simulink model "Quad_Nonlinear_Roll_PS"  (R2023a)
settings: Solver=ode4  StartTime=0.0  StopTime=0.5  FixedStep=0.02  RelTol=1e-3
values from neighbouring files (symbols this model uses):
  b = 1.10794e-5    (= 1.10794e-05)    [QuadParameter.m]    (also in Scenario_I.mat = 3.13e-05; Scenario_II.mat = 3.13e-05; final_PS.m = 3.6602e-06)
  d = 3.2e-6    (= 3.2e-06)    [QuadParameter.m]    (also in Scenario_I.mat; Scenario_II.mat)
  d_cg = 0.295    [QuadParameter.m]
  Gamma1 = Ixz*(Ixx - Iyy + Izz)/Gamma    [QuadConstants_v1.m]    (also in final_PS.m = 4.98954110218e-06)
  Gamma10 = (Ixx - Iyy)*Ixx + Ixz^2/Gamma    [QuadConstants_v1.m]    (also in final_PS.m = -1.44562619786e-05)
  Gamma11 = Ixx/Gamma    [QuadConstants_v1.m]    (also in final_PS.m = 24.4566929368)
  Gamma2 = Izz*(Izz - Iyy) + Ixz^2    [QuadConstants_v1.m]    (also in final_PS.m = 0.00290613207976)
  Gamma3 = Izz/Gamma    [QuadConstants_v1.m]    (also in final_PS.m = 42.1805100768)
  Gamma4 = Ixz/Gamma    [QuadConstants_v1.m]    (also in final_PS.m = 0.000237183411278)
  Gamma5 = I_rotor/Ixx    [QuadConstants_v1.m]    (also in final_PS.m = -0.0023457751623)
  Gamma6 = (Izz - Ixx)/Iyy    [QuadConstants_v1.m]    (also in final_PS.m = 2.52935414321)
  Gamma8 = 1/Iyy    [QuadConstants_v1.m]    (also in final_PS.m = 18.4688604257)
  Gamma9 = I_rotor/Iyy    [QuadConstants_v1.m]    (also in final_PS.m = 0.00216966508126)
  init_I = data(1, :)    [load_data.m]
  init_II = data(1, :)    [load_data.m]
  init_III = data(1, :)    [load_data.m]
  init_IV = data(1, :)    [load_data.m]
  init_V = data(1, :)    [load_data.m]
  Omega_I = Omega    [load_data.m]
  Omega_II = Omega    [load_data.m]
  Omega_III = Omega    [load_data.m]
  Omega_IV = Omega    [load_data.m]
  Omega_V = Omega    [load_data.m]
(part 1 of 2)
settings Model: Creator=Ali  LastModifiedBy=Ali
settings SolverCC: AlgebraicLoopSolver=TrustRegion
settings DebuggingCC: UnconnectedInputMsg=warning  UnconnectedOutputMsg=warning  UnconnectedLineMsg=warning
settings ModelReferenceCC: EnableRefExpFcnMdlSchedulingChecks=on

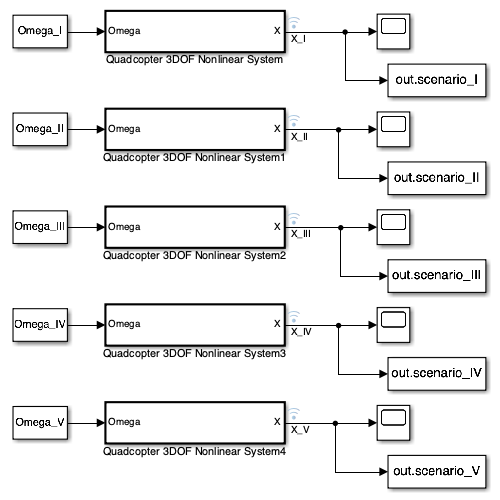
[thumbnail: Simulink's stored preview of the top-level diagram]
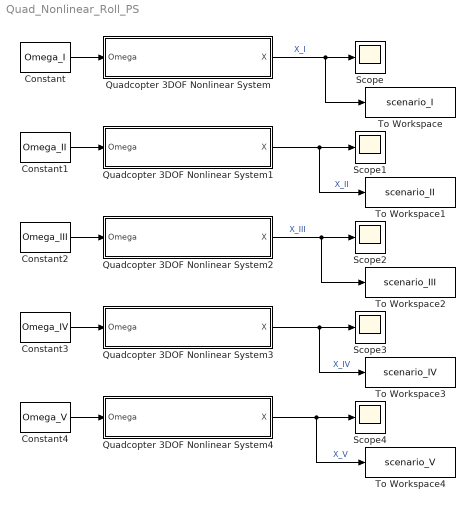
== system Quad_Nonlinear_Roll_PS ==
  Constant : Constant  Value=Omega_I
  Constant1 : Constant  Value=Omega_II
  Constant2 : Constant  Value=Omega_III
  Constant3 : Constant  Value=Omega_IV
  Constant4 : Constant  Value=Omega_V
  Quadcopter 3DOF Nonlinear System : Subsystem  TreatAsAtomicUnit=on
  Quadcopter 3DOF Nonlinear System1 : Subsystem  TreatAsAtomicUnit=on
  Quadcopter 3DOF Nonlinear System2 : Subsystem  TreatAsAtomicUnit=on
  Quadcopter 3DOF Nonlinear System3 : Subsystem  TreatAsAtomicUnit=on
  Quadcopter 3DOF Nonlinear System4 : Subsystem  TreatAsAtomicUnit=on
  Scope{,1..4} (5 alike) : Scope
  To Workspace : ToWorkspace  VariableName=scenario_I  SampleTime=-1
  To Workspace1 : ToWorkspace  VariableName=scenario_II  SampleTime=-1
  To Workspace2 : ToWorkspace  VariableName=scenario_III  SampleTime=-1
  To Workspace3 : ToWorkspace  VariableName=scenario_IV  SampleTime=-1
  To Workspace4 : ToWorkspace  VariableName=scenario_V  SampleTime=-1
  wires:
  Constant/1 -> Quadcopter 3DOF Nonlinear System/1(Omega)
  Quadcopter 3DOF Nonlinear System/1(X) -> To Workspace/1, Scope/1  "X_I"
  Quadcopter 3DOF Nonlinear System1/1(X) -> To Workspace1/1, Scope1/1  "X_II"
  Constant1/1 -> Quadcopter 3DOF Nonlinear System1/1(Omega)
  Quadcopter 3DOF Nonlinear System2/1(X) -> To Workspace2/1, Scope2/1  "X_III"
  Constant2/1 -> Quadcopter 3DOF Nonlinear System2/1(Omega)
  Quadcopter 3DOF Nonlinear System3/1(X) -> To Workspace3/1, Scope3/1  "X_IV"
  Constant3/1 -> Quadcopter 3DOF Nonlinear System3/1(Omega)
  Quadcopter 3DOF Nonlinear System4/1(X) -> To Workspace4/1, Scope4/1  "X_V"
  Constant4/1 -> Quadcopter 3DOF Nonlinear System4/1(Omega)

== system Quad_Nonlinear_Roll_PS/Quadcopter 3DOF Nonlinear System ==
  Omega : Inport
  Integrator : Integrator  InitialCondition=init_I
  Quad System : Subsystem
  X : Outport
  wires:
  Integrator/1 -> Quad System/1(X), X/1  "X"
  Quad System/1(dot(X)) -> Integrator/1  "dot(X)"
  Omega/1 -> Quad System/2(Omega)

== system Quad_Nonlinear_Roll_PS/Quadcopter 3DOF Nonlinear System1 ==
  Omega : Inport
  Integrator : Integrator  InitialCondition=init_II
  Quad System : Subsystem
  X : Outport
  wires:
  Integrator/1 -> Quad System/1(X), X/1  "X"
  Quad System/1(dot(X)) -> Integrator/1  "dot(X)"
  Omega/1 -> Quad System/2(Omega)

== system Quad_Nonlinear_Roll_PS/Quadcopter 3DOF Nonlinear System2 ==
  Omega : Inport
  Integrator : Integrator  InitialCondition=init_III
  Quad System : Subsystem
  X : Outport
  wires:
  Integrator/1 -> Quad System/1(X), X/1  "X"
  Quad System/1(dot(X)) -> Integrator/1  "dot(X)"
  Omega/1 -> Quad System/2(Omega)

== system Quad_Nonlinear_Roll_PS/Quadcopter 3DOF Nonlinear System3 ==
  Omega : Inport
  Integrator : Integrator  InitialCondition=init_IV
  Quad System : Subsystem
  X : Outport
  wires:
  Integrator/1 -> Quad System/1(X), X/1  "X"
  Quad System/1(dot(X)) -> Integrator/1  "dot(X)"
  Omega/1 -> Quad System/2(Omega)

== system Quad_Nonlinear_Roll_PS/Quadcopter 3DOF Nonlinear System4 ==
  Omega : Inport
  Integrator : Integrator  InitialCondition=init_V
  Quad System : Subsystem
  X : Outport
  wires:
  Integrator/1 -> Quad System/1(X), X/1  "X"
  Quad System/1(dot(X)) -> Integrator/1  "dot(X)"
  Omega/1 -> Quad System/2(Omega)

== system Quad_Nonlinear_Roll_PS/Quadcopter 3DOF Nonlinear System/Quad System ==
  X : Inport
  Omega : Inport  Port=2
  Quad System : Subsystem
  Selector : Selector  InputPortWidth=6  IndexOptions=Index vector (dialog)  Indices=[1 4]  OutputSizes=1
  Subsystem : Subsystem
  dot(X) : Outport
  wires:
  Selector/1 -> dot(X)/1  "dot(X)"
  X/1 -> Subsystem/1(X)
  Omega/1 -> Quad System/2(Omega)
  Quad System/1(dot(X)) -> Selector/1  "dot(X)"
  Subsystem/1(X_6) -> Quad System/1(X)

== system Quad_Nonlinear_Roll_PS/Quadcopter 3DOF Nonlinear System1/Quad System ==
  X : Inport
  Omega : Inport  Port=2
  Quad System : Subsystem
  Selector : Selector  InputPortWidth=6  IndexOptions=Index vector (dialog)  Indices=[1 4]  OutputSizes=1
  Subsystem : Subsystem
  dot(X) : Outport
  wires:
  Selector/1 -> dot(X)/1  "dot(X)"
  X/1 -> Subsystem/1(X)
  Omega/1 -> Quad System/2(Omega)
  Quad System/1(dot(X)) -> Selector/1  "dot(X)"
  Subsystem/1(X_6) -> Quad System/1(X)

== system Quad_Nonlinear_Roll_PS/Quadcopter 3DOF Nonlinear System2/Quad System ==
  X : Inport
  Omega : Inport  Port=2
  Quad System : Subsystem
  Selector : Selector  InputPortWidth=6  IndexOptions=Index vector (dialog)  Indices=[1 4]  OutputSizes=1
  Subsystem : Subsystem
  dot(X) : Outport
  wires:
  Selector/1 -> dot(X)/1  "dot(X)"
  X/1 -> Subsystem/1(X)
  Omega/1 -> Quad System/2(Omega)
  Quad System/1(dot(X)) -> Selector/1  "dot(X)"
  Subsystem/1(X_6) -> Quad System/1(X)

== system Quad_Nonlinear_Roll_PS/Quadcopter 3DOF Nonlinear System3/Quad System ==
  X : Inport
  Omega : Inport  Port=2
  Quad System : Subsystem
  Selector : Selector  InputPortWidth=6  IndexOptions=Index vector (dialog)  Indices=[1 4]  OutputSizes=1
  Subsystem : Subsystem
  dot(X) : Outport
  wires:
  Selector/1 -> dot(X)/1  "dot(X)"
  X/1 -> Subsystem/1(X)
  Omega/1 -> Quad System/2(Omega)
  Quad System/1(dot(X)) -> Selector/1  "dot(X)"
  Subsystem/1(X_6) -> Quad System/1(X)

== system Quad_Nonlinear_Roll_PS/Quadcopter 3DOF Nonlinear System4/Quad System ==
  X : Inport
  Omega : Inport  Port=2
  Quad System : Subsystem
  Selector : Selector  InputPortWidth=6  IndexOptions=Index vector (dialog)  Indices=[1 4]  OutputSizes=1
  Subsystem : Subsystem
  dot(X) : Outport
  wires:
  Selector/1 -> dot(X)/1  "dot(X)"
  X/1 -> Subsystem/1(X)
  Omega/1 -> Quad System/2(Omega)
  Quad System/1(dot(X)) -> Selector/1  "dot(X)"
  Subsystem/1(X_6) -> Quad System/1(X)

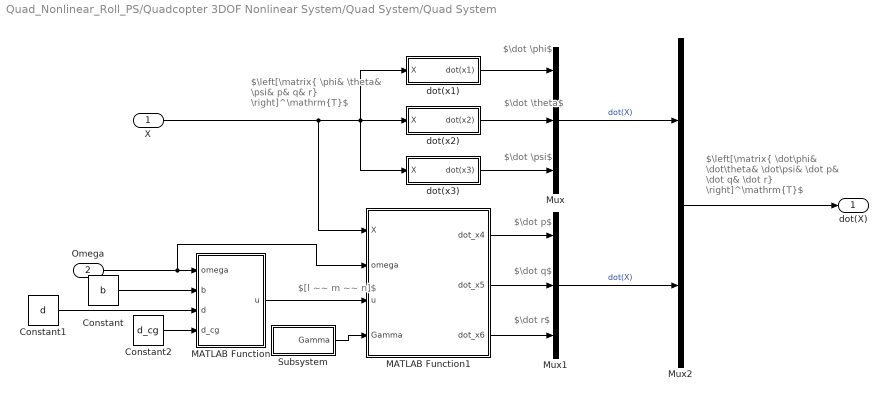
== system Quad_Nonlinear_Roll_PS/Quadcopter 3DOF Nonlinear System/Quad System/Quad System ==
  note: $\dot \phi$
  note: $\left[\matrix{ \phi& \theta& \psi& p& q& r} \right]^\mathrm{T}$
  note: $[l ~~ m ~~ n]$
  note: $\dot \theta$
  note: $\dot \psi$
  note: $\dot p$
  note: $\dot q$
  note: $\dot r$
  note: $\left[\matrix{ \dot\phi& \dot\theta& \dot\psi& \dot p& \dot q& \dot r} \right]^\mathrm{T}$
  X : Inport
  Omega : Inport  Port=2
  Constant : Constant  Value=b
  Constant1 : Constant  Value=d
  Constant2 : Constant  Value=d_cg
  MATLAB Function : MATLAB Function  TreatAsAtomicUnit=on
  MATLAB Function1 : MATLAB Function  TreatAsAtomicUnit=on
  Mux : Mux  Inputs=3
  Mux1 : Mux  Inputs=3
  Mux2 : Mux  Inputs=2
  Subsystem : Subsystem
  dot(x1) : Subsystem
  dot(x2) : Subsystem
  dot(x3) : Subsystem
  dot(X) : Outport
  wires:
  X/1 -> MATLAB Function1/1(X), dot(x3)/1(X), dot(x1)/1(X), dot(x2)/1(X)
  Omega/1 -> MATLAB Function1/2(omega), MATLAB Function/1(omega)
  MATLAB Function1/2(dot_x5) -> Mux1/2
  dot(x2)/1(dot(x2)) -> Mux/2
  MATLAB Function1/1(dot_x4) -> Mux1/1
  dot(x3)/1(dot(x3)) -> Mux/3
  dot(x1)/1(dot(x1)) -> Mux/1
  MATLAB Function1/3(dot_x6) -> Mux1/3
  Constant/1 -> MATLAB Function/2(b)
  Constant1/1 -> MATLAB Function/3(d)
  MATLAB Function/1(u) -> MATLAB Function1/3(u)
  Mux1/1 -> Mux2/2  "dot(X)"
  Mux/1 -> Mux2/1  "dot(X)"
  Mux2/1 -> dot(X)/1
  Subsystem/1(Gamma) -> MATLAB Function1/4(Gamma)
  Constant2/1 -> MATLAB Function/4(d_cg)

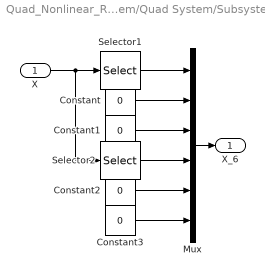
== system Quad_Nonlinear_Roll_PS/Quadcopter 3DOF Nonlinear System/Quad System/Subsystem ==
  X : Inport
  Constant{,1..3} (4 alike) : Constant  Value=0
  Mux : Mux  Inputs=6
  Selector1 : Selector  InputPortWidth=2  IndexOptions=Index vector (dialog)  Indices=[1]  OutputSizes=1
  Selector2 : Selector  InputPortWidth=2  IndexOptions=Index vector (dialog)  Indices=[2]  OutputSizes=1
  X_6 : Outport
  wires:
  Constant3/1 -> Mux/6
  Constant1/1 -> Mux/3
  Mux/1 -> X_6/1
  Constant/1 -> Mux/2
  Selector2/1 -> Mux/4
  Selector1/1 -> Mux/1
  Constant2/1 -> Mux/5
  X/1 -> Selector2/1, Selector1/1

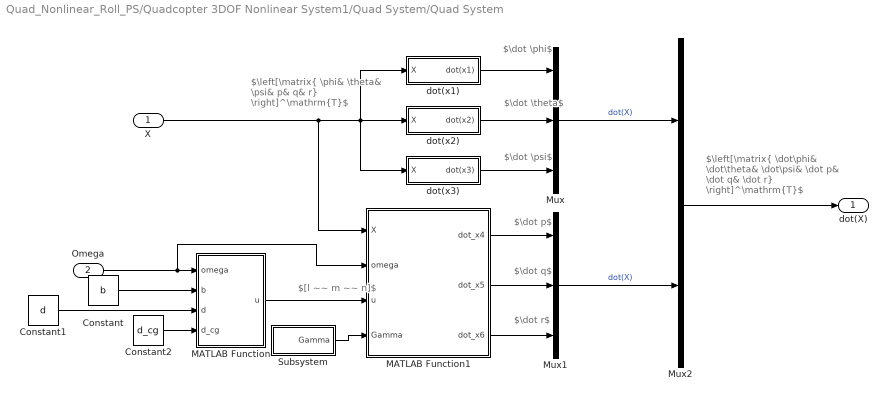
== system Quad_Nonlinear_Roll_PS/Quadcopter 3DOF Nonlinear System1/Quad System/Quad System ==
  note: $\dot \phi$
  note: $\left[\matrix{ \phi& \theta& \psi& p& q& r} \right]^\mathrm{T}$
  note: $[l ~~ m ~~ n]$
  note: $\dot \theta$
  note: $\dot \psi$
  note: $\dot p$
  note: $\dot q$
  note: $\dot r$
  note: $\left[\matrix{ \dot\phi& \dot\theta& \dot\psi& \dot p& \dot q& \dot r} \right]^\mathrm{T}$
  X : Inport
  Omega : Inport  Port=2
  Constant : Constant  Value=b
  Constant1 : Constant  Value=d
  Constant2 : Constant  Value=d_cg
  MATLAB Function : MATLAB Function  TreatAsAtomicUnit=on
  MATLAB Function1 : MATLAB Function  TreatAsAtomicUnit=on
  Mux : Mux  Inputs=3
  Mux1 : Mux  Inputs=3
  Mux2 : Mux  Inputs=2
  Subsystem : Subsystem
  dot(x1) : Subsystem
  dot(x2) : Subsystem
  dot(x3) : Subsystem
  dot(X) : Outport
  wires:
  X/1 -> MATLAB Function1/1(X), dot(x3)/1(X), dot(x1)/1(X), dot(x2)/1(X)
  Omega/1 -> MATLAB Function1/2(omega), MATLAB Function/1(omega)
  MATLAB Function1/2(dot_x5) -> Mux1/2
  dot(x2)/1(dot(x2)) -> Mux/2
  MATLAB Function1/1(dot_x4) -> Mux1/1
  dot(x3)/1(dot(x3)) -> Mux/3
  dot(x1)/1(dot(x1)) -> Mux/1
  MATLAB Function1/3(dot_x6) -> Mux1/3
  Constant/1 -> MATLAB Function/2(b)
  Constant1/1 -> MATLAB Function/3(d)
  MATLAB Function/1(u) -> MATLAB Function1/3(u)
  Mux1/1 -> Mux2/2  "dot(X)"
  Mux/1 -> Mux2/1  "dot(X)"
  Mux2/1 -> dot(X)/1
  Subsystem/1(Gamma) -> MATLAB Function1/4(Gamma)
  Constant2/1 -> MATLAB Function/4(d_cg)

== system Quad_Nonlinear_Roll_PS/Quadcopter 3DOF Nonlinear System1/Quad System/Subsystem ==
  X : Inport
  Constant{,1..3} (4 alike) : Constant  Value=0
  Mux : Mux  Inputs=6
  Selector1 : Selector  InputPortWidth=2  IndexOptions=Index vector (dialog)  Indices=[1]  OutputSizes=1
  Selector2 : Selector  InputPortWidth=2  IndexOptions=Index vector (dialog)  Indices=[2]  OutputSizes=1
  X_6 : Outport
  wires:
  Constant3/1 -> Mux/6
  Constant1/1 -> Mux/3
  Mux/1 -> X_6/1
  Constant/1 -> Mux/2
  Selector2/1 -> Mux/4
  Selector1/1 -> Mux/1
  Constant2/1 -> Mux/5
  X/1 -> Selector2/1, Selector1/1

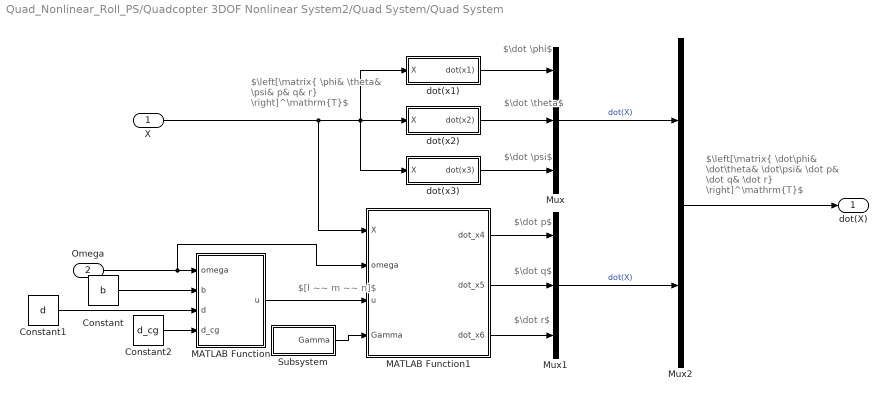
== system Quad_Nonlinear_Roll_PS/Quadcopter 3DOF Nonlinear System2/Quad System/Quad System ==
  note: $\dot \phi$
  note: $\left[\matrix{ \phi& \theta& \psi& p& q& r} \right]^\mathrm{T}$
  note: $[l ~~ m ~~ n]$
  note: $\dot \theta$
  note: $\dot \psi$
  note: $\dot p$
  note: $\dot q$
  note: $\dot r$
  note: $\left[\matrix{ \dot\phi& \dot\theta& \dot\psi& \dot p& \dot q& \dot r} \right]^\mathrm{T}$
  X : Inport
  Omega : Inport  Port=2
  Constant : Constant  Value=b
  Constant1 : Constant  Value=d
  Constant2 : Constant  Value=d_cg
  MATLAB Function : MATLAB Function  TreatAsAtomicUnit=on
  MATLAB Function1 : MATLAB Function  TreatAsAtomicUnit=on
  Mux : Mux  Inputs=3
  Mux1 : Mux  Inputs=3
  Mux2 : Mux  Inputs=2
  Subsystem : Subsystem
  dot(x1) : Subsystem
  dot(x2) : Subsystem
  dot(x3) : Subsystem
  dot(X) : Outport
  wires:
  X/1 -> MATLAB Function1/1(X), dot(x3)/1(X), dot(x1)/1(X), dot(x2)/1(X)
  Omega/1 -> MATLAB Function1/2(omega), MATLAB Function/1(omega)
  MATLAB Function1/2(dot_x5) -> Mux1/2
  dot(x2)/1(dot(x2)) -> Mux/2
  MATLAB Function1/1(dot_x4) -> Mux1/1
  dot(x3)/1(dot(x3)) -> Mux/3
  dot(x1)/1(dot(x1)) -> Mux/1
  MATLAB Function1/3(dot_x6) -> Mux1/3
  Constant/1 -> MATLAB Function/2(b)
  Constant1/1 -> MATLAB Function/3(d)
  MATLAB Function/1(u) -> MATLAB Function1/3(u)
  Mux1/1 -> Mux2/2  "dot(X)"
  Mux/1 -> Mux2/1  "dot(X)"
  Mux2/1 -> dot(X)/1
  Subsystem/1(Gamma) -> MATLAB Function1/4(Gamma)
  Constant2/1 -> MATLAB Function/4(d_cg)

== system Quad_Nonlinear_Roll_PS/Quadcopter 3DOF Nonlinear System2/Quad System/Subsystem ==
  X : Inport
  Constant{,1..3} (4 alike) : Constant  Value=0
  Mux : Mux  Inputs=6
  Selector1 : Selector  InputPortWidth=2  IndexOptions=Index vector (dialog)  Indices=[1]  OutputSizes=1
  Selector2 : Selector  InputPortWidth=2  IndexOptions=Index vector (dialog)  Indices=[2]  OutputSizes=1
  X_6 : Outport
  wires:
  Constant3/1 -> Mux/6
  Constant1/1 -> Mux/3
  Mux/1 -> X_6/1
  Constant/1 -> Mux/2
  Selector2/1 -> Mux/4
  Selector1/1 -> Mux/1
  Constant2/1 -> Mux/5
  X/1 -> Selector2/1, Selector1/1

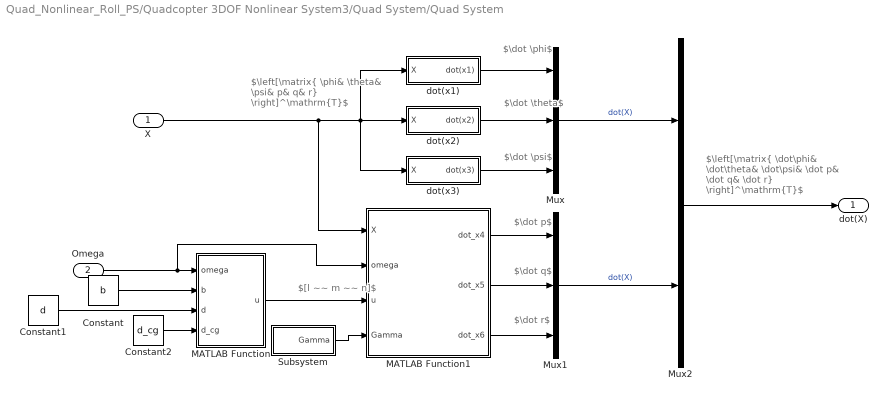
== system Quad_Nonlinear_Roll_PS/Quadcopter 3DOF Nonlinear System3/Quad System/Quad System ==
  note: $\dot \phi$
  note: $\left[\matrix{ \phi& \theta& \psi& p& q& r} \right]^\mathrm{T}$
  note: $[l ~~ m ~~ n]$
  note: $\dot \theta$
  note: $\dot \psi$
  note: $\dot p$
  note: $\dot q$
  note: $\dot r$
  note: $\left[\matrix{ \dot\phi& \dot\theta& \dot\psi& \dot p& \dot q& \dot r} \right]^\mathrm{T}$
  X : Inport
  Omega : Inport  Port=2
  Constant : Constant  Value=b
  Constant1 : Constant  Value=d
  Constant2 : Constant  Value=d_cg
  MATLAB Function : MATLAB Function  TreatAsAtomicUnit=on
  MATLAB Function1 : MATLAB Function  TreatAsAtomicUnit=on
  Mux : Mux  Inputs=3
  Mux1 : Mux  Inputs=3
  Mux2 : Mux  Inputs=2
  Subsystem : Subsystem
  dot(x1) : Subsystem
  dot(x2) : Subsystem
  dot(x3) : Subsystem
  dot(X) : Outport
  wires:
  X/1 -> MATLAB Function1/1(X), dot(x3)/1(X), dot(x1)/1(X), dot(x2)/1(X)
  Omega/1 -> MATLAB Function1/2(omega), MATLAB Function/1(omega)
  MATLAB Function1/2(dot_x5) -> Mux1/2
  dot(x2)/1(dot(x2)) -> Mux/2
  MATLAB Function1/1(dot_x4) -> Mux1/1
  dot(x3)/1(dot(x3)) -> Mux/3
  dot(x1)/1(dot(x1)) -> Mux/1
  MATLAB Function1/3(dot_x6) -> Mux1/3
  Constant/1 -> MATLAB Function/2(b)
  Constant1/1 -> MATLAB Function/3(d)
  MATLAB Function/1(u) -> MATLAB Function1/3(u)
  Mux1/1 -> Mux2/2  "dot(X)"
  Mux/1 -> Mux2/1  "dot(X)"
  Mux2/1 -> dot(X)/1
  Subsystem/1(Gamma) -> MATLAB Function1/4(Gamma)
  Constant2/1 -> MATLAB Function/4(d_cg)

== system Quad_Nonlinear_Roll_PS/Quadcopter 3DOF Nonlinear System3/Quad System/Subsystem ==
  X : Inport
  Constant{,1..3} (4 alike) : Constant  Value=0
  Mux : Mux  Inputs=6
  Selector1 : Selector  InputPortWidth=2  IndexOptions=Index vector (dialog)  Indices=[1]  OutputSizes=1
  Selector2 : Selector  InputPortWidth=2  IndexOptions=Index vector (dialog)  Indices=[2]  OutputSizes=1
  X_6 : Outport
  wires:
  Constant3/1 -> Mux/6
  Constant1/1 -> Mux/3
  Mux/1 -> X_6/1
  Constant/1 -> Mux/2
  Selector2/1 -> Mux/4
  Selector1/1 -> Mux/1
  Constant2/1 -> Mux/5
  X/1 -> Selector2/1, Selector1/1

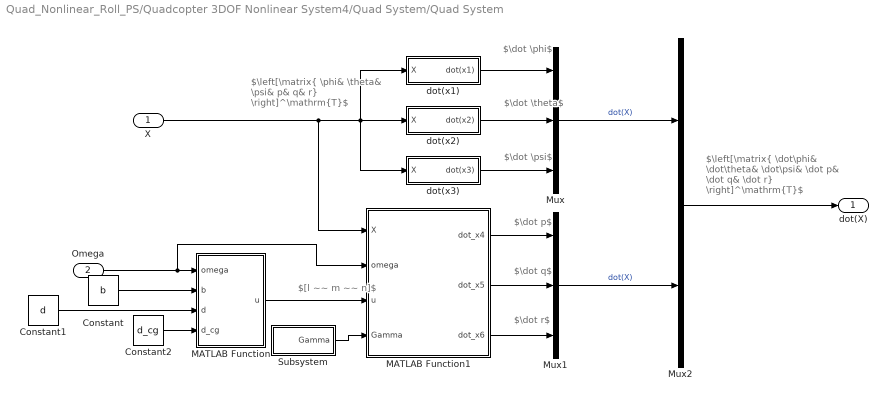
== system Quad_Nonlinear_Roll_PS/Quadcopter 3DOF Nonlinear System4/Quad System/Quad System ==
  note: $\dot \phi$
  note: $\left[\matrix{ \phi& \theta& \psi& p& q& r} \right]^\mathrm{T}$
  note: $[l ~~ m ~~ n]$
  note: $\dot \theta$
  note: $\dot \psi$
  note: $\dot p$
  note: $\dot q$
  note: $\dot r$
  note: $\left[\matrix{ \dot\phi& \dot\theta& \dot\psi& \dot p& \dot q& \dot r} \right]^\mathrm{T}$
  X : Inport
  Omega : Inport  Port=2
  Constant : Constant  Value=b
  Constant1 : Constant  Value=d
  Constant2 : Constant  Value=d_cg
  MATLAB Function : MATLAB Function  TreatAsAtomicUnit=on
  MATLAB Function1 : MATLAB Function  TreatAsAtomicUnit=on
  Mux : Mux  Inputs=3
  Mux1 : Mux  Inputs=3
  Mux2 : Mux  Inputs=2
  Subsystem : Subsystem
  dot(x1) : Subsystem
  dot(x2) : Subsystem
  dot(x3) : Subsystem
  dot(X) : Outport
  wires:
  X/1 -> MATLAB Function1/1(X), dot(x3)/1(X), dot(x1)/1(X), dot(x2)/1(X)
  Omega/1 -> MATLAB Function1/2(omega), MATLAB Function/1(omega)
  MATLAB Function1/2(dot_x5) -> Mux1/2
  dot(x2)/1(dot(x2)) -> Mux/2
  MATLAB Function1/1(dot_x4) -> Mux1/1
  dot(x3)/1(dot(x3)) -> Mux/3
  dot(x1)/1(dot(x1)) -> Mux/1
  MATLAB Function1/3(dot_x6) -> Mux1/3
  Constant/1 -> MATLAB Function/2(b)
  Constant1/1 -> MATLAB Function/3(d)
  MATLAB Function/1(u) -> MATLAB Function1/3(u)
  Mux1/1 -> Mux2/2  "dot(X)"
  Mux/1 -> Mux2/1  "dot(X)"
  Mux2/1 -> dot(X)/1
  Subsystem/1(Gamma) -> MATLAB Function1/4(Gamma)
  Constant2/1 -> MATLAB Function/4(d_cg)

== system Quad_Nonlinear_Roll_PS/Quadcopter 3DOF Nonlinear System4/Quad System/Subsystem ==
  X : Inport
  Constant{,1..3} (4 alike) : Constant  Value=0
  Mux : Mux  Inputs=6
  Selector1 : Selector  InputPortWidth=2  IndexOptions=Index vector (dialog)  Indices=[1]  OutputSizes=1
  Selector2 : Selector  InputPortWidth=2  IndexOptions=Index vector (dialog)  Indices=[2]  OutputSizes=1
  X_6 : Outport
  wires:
  Constant3/1 -> Mux/6
  Constant1/1 -> Mux/3
  Mux/1 -> X_6/1
  Constant/1 -> Mux/2
  Selector2/1 -> Mux/4
  Selector1/1 -> Mux/1
  Constant2/1 -> Mux/5
  X/1 -> Selector2/1, Selector1/1

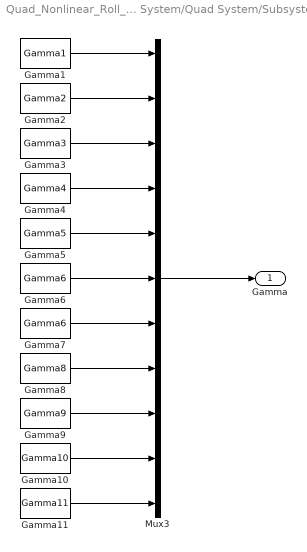
== system Quad_Nonlinear_Roll_PS/Quadcopter 3DOF Nonlinear System/Quad System/Quad System/Subsystem ==
  Gamma1 : Constant  Value=Gamma1
  Gamma10 : Constant  Value=Gamma10
  Gamma11 : Constant  Value=Gamma11
  Gamma2 : Constant  Value=Gamma2
  Gamma3 : Constant  Value=Gamma3
  Gamma4 : Constant  Value=Gamma4
  Gamma5 : Constant  Value=Gamma5
  Gamma6 : Constant  Value=Gamma6
  Gamma7 : Constant  Value=Gamma6
  Gamma8 : Constant  Value=Gamma8
  Gamma9 : Constant  Value=Gamma9
  Mux3 : Mux  Inputs=11
  Gamma : Outport
  wires:
  Gamma9/1 -> Mux3/9
  Gamma6/1 -> Mux3/6
  Mux3/1 -> Gamma/1
  Gamma8/1 -> Mux3/8
  Gamma5/1 -> Mux3/5
  Gamma7/1 -> Mux3/7
  Gamma4/1 -> Mux3/4
  Gamma3/1 -> Mux3/3
  Gamma2/1 -> Mux3/2
  Gamma1/1 -> Mux3/1
  Gamma10/1 -> Mux3/10
  Gamma11/1 -> Mux3/11

== system Quad_Nonlinear_Roll_PS/Quadcopter 3DOF Nonlinear System/Quad System/Quad System/dot(x1) ==
  X : Inport
  1 : Subsystem
  Add : Sum  Inputs=+++
  Subsystem : Subsystem
  Subsystem1 : Subsystem
  dot(x1) : Outport
  wires:
  X/1 -> Subsystem1/1(X), Subsystem/1(X), 1/1(X)  "X"
  Subsystem1/1(x4) -> Add/3
  Subsystem/1(x6cos(x1)tan(x2)) -> Add/2
  Add/1 -> dot(x1)/1
  1/1(x5sin(x1)tan(x2)) -> Add/1

== system Quad_Nonlinear_Roll_PS/Quadcopter 3DOF Nonlinear System/Quad System/Quad System/dot(x2) ==
  X : Inport
  1 : Subsystem
  Add : Sum  Inputs=+-
  Subsystem : Subsystem
  dot(x2) : Outport
  wires:
  X/1 -> Subsystem/1(X), 1/1(X)  "X"
  Subsystem/1(x6sin(x1)) -> Add/2
  Add/1 -> dot(x2)/1
  1/1(x5cos(x1)) -> Add/1

== system Quad_Nonlinear_Roll_PS/Quadcopter 3DOF Nonlinear System/Quad System/Quad System/dot(x3) ==
  X : Inport
  1 : Subsystem
  Add : Sum
  Product : Product
  Subsystem : Subsystem
  Subsystem1 : Subsystem
  dot(x3) : Outport
  wires:
  X/1 -> Subsystem1/1(X), Subsystem/1(X), 1/1(X)  "X"
  Subsystem/1(x6cos(x1)) -> Add/2
  1/1(x5sin(x1)) -> Add/1
  Product/1 -> dot(x3)/1
  Add/1 -> Product/1
  Subsystem1/1(sec(x2)) -> Product/2

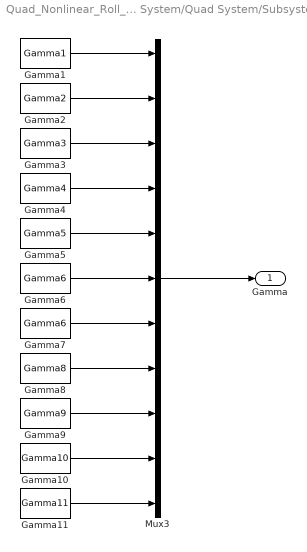
== system Quad_Nonlinear_Roll_PS/Quadcopter 3DOF Nonlinear System1/Quad System/Quad System/Subsystem ==
  Gamma1 : Constant  Value=Gamma1
  Gamma10 : Constant  Value=Gamma10
  Gamma11 : Constant  Value=Gamma11
  Gamma2 : Constant  Value=Gamma2
  Gamma3 : Constant  Value=Gamma3
  Gamma4 : Constant  Value=Gamma4
  Gamma5 : Constant  Value=Gamma5
  Gamma6 : Constant  Value=Gamma6
  Gamma7 : Constant  Value=Gamma6
  Gamma8 : Constant  Value=Gamma8
  Gamma9 : Constant  Value=Gamma9
  Mux3 : Mux  Inputs=11
  Gamma : Outport
  wires:
  Gamma9/1 -> Mux3/9
  Gamma6/1 -> Mux3/6
  Mux3/1 -> Gamma/1
  Gamma8/1 -> Mux3/8
  Gamma5/1 -> Mux3/5
  Gamma7/1 -> Mux3/7
  Gamma4/1 -> Mux3/4
  Gamma3/1 -> Mux3/3
  Gamma2/1 -> Mux3/2
  Gamma1/1 -> Mux3/1
  Gamma10/1 -> Mux3/10
  Gamma11/1 -> Mux3/11

== system Quad_Nonlinear_Roll_PS/Quadcopter 3DOF Nonlinear System1/Quad System/Quad System/dot(x1) ==
  X : Inport
  1 : Subsystem
  Add : Sum  Inputs=+++
  Subsystem : Subsystem
  Subsystem1 : Subsystem
  dot(x1) : Outport
  wires:
  X/1 -> Subsystem1/1(X), Subsystem/1(X), 1/1(X)  "X"
  Subsystem1/1(x4) -> Add/3
  Subsystem/1(x6cos(x1)tan(x2)) -> Add/2
  Add/1 -> dot(x1)/1
  1/1(x5sin(x1)tan(x2)) -> Add/1

== system Quad_Nonlinear_Roll_PS/Quadcopter 3DOF Nonlinear System1/Quad System/Quad System/dot(x2) ==
  X : Inport
  1 : Subsystem
  Add : Sum  Inputs=+-
  Subsystem : Subsystem
  dot(x2) : Outport
  wires:
  X/1 -> Subsystem/1(X), 1/1(X)  "X"
  Subsystem/1(x6sin(x1)) -> Add/2
  Add/1 -> dot(x2)/1
  1/1(x5cos(x1)) -> Add/1

== system Quad_Nonlinear_Roll_PS/Quadcopter 3DOF Nonlinear System1/Quad System/Quad System/dot(x3) ==
  X : Inport
  1 : Subsystem
  Add : Sum
  Product : Product
  Subsystem : Subsystem
  Subsystem1 : Subsystem
  dot(x3) : Outport
  wires:
  X/1 -> Subsystem1/1(X), Subsystem/1(X), 1/1(X)  "X"
  Subsystem/1(x6cos(x1)) -> Add/2
  1/1(x5sin(x1)) -> Add/1
  Product/1 -> dot(x3)/1
  Add/1 -> Product/1
  Subsystem1/1(sec(x2)) -> Product/2

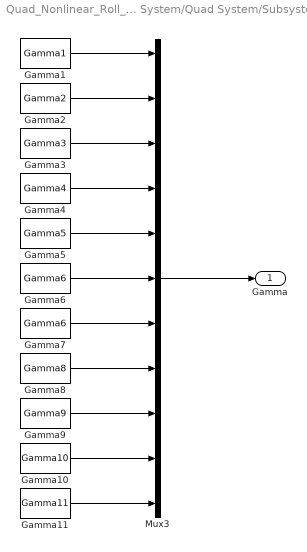
== system Quad_Nonlinear_Roll_PS/Quadcopter 3DOF Nonlinear System2/Quad System/Quad System/Subsystem ==
  Gamma1 : Constant  Value=Gamma1
  Gamma10 : Constant  Value=Gamma10
  Gamma11 : Constant  Value=Gamma11
  Gamma2 : Constant  Value=Gamma2
  Gamma3 : Constant  Value=Gamma3
  Gamma4 : Constant  Value=Gamma4
  Gamma5 : Constant  Value=Gamma5
  Gamma6 : Constant  Value=Gamma6
  Gamma7 : Constant  Value=Gamma6
  Gamma8 : Constant  Value=Gamma8
  Gamma9 : Constant  Value=Gamma9
  Mux3 : Mux  Inputs=11
  Gamma : Outport
  wires:
  Gamma9/1 -> Mux3/9
  Gamma6/1 -> Mux3/6
  Mux3/1 -> Gamma/1
  Gamma8/1 -> Mux3/8
  Gamma5/1 -> Mux3/5
  Gamma7/1 -> Mux3/7
  Gamma4/1 -> Mux3/4
  Gamma3/1 -> Mux3/3
  Gamma2/1 -> Mux3/2
  Gamma1/1 -> Mux3/1
  Gamma10/1 -> Mux3/10
  Gamma11/1 -> Mux3/11

== system Quad_Nonlinear_Roll_PS/Quadcopter 3DOF Nonlinear System2/Quad System/Quad System/dot(x1) ==
  X : Inport
  1 : Subsystem
  Add : Sum  Inputs=+++
  Subsystem : Subsystem
  Subsystem1 : Subsystem
  dot(x1) : Outport
  wires:
  X/1 -> Subsystem1/1(X), Subsystem/1(X), 1/1(X)  "X"
  Subsystem1/1(x4) -> Add/3
  Subsystem/1(x6cos(x1)tan(x2)) -> Add/2
  Add/1 -> dot(x1)/1
  1/1(x5sin(x1)tan(x2)) -> Add/1

== system Quad_Nonlinear_Roll_PS/Quadcopter 3DOF Nonlinear System2/Quad System/Quad System/dot(x2) ==
  X : Inport
  1 : Subsystem
  Add : Sum  Inputs=+-
  Subsystem : Subsystem
  dot(x2) : Outport
  wires:
  X/1 -> Subsystem/1(X), 1/1(X)  "X"
  Subsystem/1(x6sin(x1)) -> Add/2
  Add/1 -> dot(x2)/1
  1/1(x5cos(x1)) -> Add/1

== system Quad_Nonlinear_Roll_PS/Quadcopter 3DOF Nonlinear System2/Quad System/Quad System/dot(x3) ==
  X : Inport
  1 : Subsystem
  Add : Sum
  Product : Product
  Subsystem : Subsystem
  Subsystem1 : Subsystem
  dot(x3) : Outport
  wires:
  X/1 -> Subsystem1/1(X), Subsystem/1(X), 1/1(X)  "X"
  Subsystem/1(x6cos(x1)) -> Add/2
  1/1(x5sin(x1)) -> Add/1
  Product/1 -> dot(x3)/1
  Add/1 -> Product/1
  Subsystem1/1(sec(x2)) -> Product/2

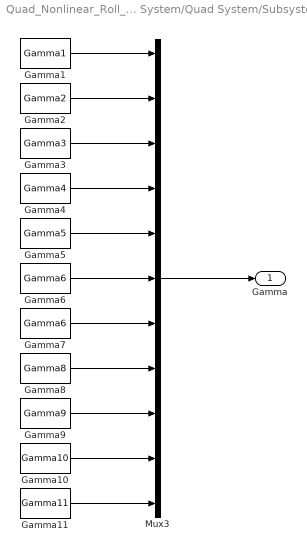
== system Quad_Nonlinear_Roll_PS/Quadcopter 3DOF Nonlinear System3/Quad System/Quad System/Subsystem ==
  Gamma1 : Constant  Value=Gamma1
  Gamma10 : Constant  Value=Gamma10
  Gamma11 : Constant  Value=Gamma11
  Gamma2 : Constant  Value=Gamma2
  Gamma3 : Constant  Value=Gamma3
  Gamma4 : Constant  Value=Gamma4
  Gamma5 : Constant  Value=Gamma5
  Gamma6 : Constant  Value=Gamma6
  Gamma7 : Constant  Value=Gamma6
  Gamma8 : Constant  Value=Gamma8
  Gamma9 : Constant  Value=Gamma9
  Mux3 : Mux  Inputs=11
  Gamma : Outport
  wires:
  Gamma9/1 -> Mux3/9
  Gamma6/1 -> Mux3/6
  Mux3/1 -> Gamma/1
  Gamma8/1 -> Mux3/8
  Gamma5/1 -> Mux3/5
  Gamma7/1 -> Mux3/7
  Gamma4/1 -> Mux3/4
  Gamma3/1 -> Mux3/3
  Gamma2/1 -> Mux3/2
  Gamma1/1 -> Mux3/1
  Gamma10/1 -> Mux3/10
  Gamma11/1 -> Mux3/11

== system Quad_Nonlinear_Roll_PS/Quadcopter 3DOF Nonlinear System3/Quad System/Quad System/dot(x1) ==
  X : Inport
  1 : Subsystem
  Add : Sum  Inputs=+++
  Subsystem : Subsystem
  Subsystem1 : Subsystem
  dot(x1) : Outport
  wires:
  X/1 -> Subsystem1/1(X), Subsystem/1(X), 1/1(X)  "X"
  Subsystem1/1(x4) -> Add/3
  Subsystem/1(x6cos(x1)tan(x2)) -> Add/2
  Add/1 -> dot(x1)/1
  1/1(x5sin(x1)tan(x2)) -> Add/1

== system Quad_Nonlinear_Roll_PS/Quadcopter 3DOF Nonlinear System3/Quad System/Quad System/dot(x2) ==
  X : Inport
  1 : Subsystem
  Add : Sum  Inputs=+-
  Subsystem : Subsystem
  dot(x2) : Outport
  wires:
  X/1 -> Subsystem/1(X), 1/1(X)  "X"
  Subsystem/1(x6sin(x1)) -> Add/2
  Add/1 -> dot(x2)/1
  1/1(x5cos(x1)) -> Add/1

== system Quad_Nonlinear_Roll_PS/Quadcopter 3DOF Nonlinear System3/Quad System/Quad System/dot(x3) ==
  X : Inport
  1 : Subsystem
  Add : Sum
  Product : Product
  Subsystem : Subsystem
  Subsystem1 : Subsystem
  dot(x3) : Outport
  wires:
  X/1 -> Subsystem1/1(X), Subsystem/1(X), 1/1(X)  "X"
  Subsystem/1(x6cos(x1)) -> Add/2
  1/1(x5sin(x1)) -> Add/1
  Product/1 -> dot(x3)/1
  Add/1 -> Product/1
  Subsystem1/1(sec(x2)) -> Product/2

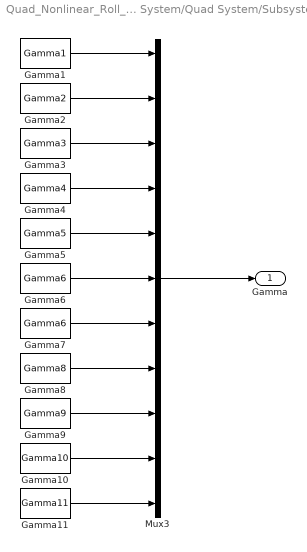
== system Quad_Nonlinear_Roll_PS/Quadcopter 3DOF Nonlinear System4/Quad System/Quad System/Subsystem ==
  Gamma1 : Constant  Value=Gamma1
  Gamma10 : Constant  Value=Gamma10
  Gamma11 : Constant  Value=Gamma11
  Gamma2 : Constant  Value=Gamma2
  Gamma3 : Constant  Value=Gamma3
  Gamma4 : Constant  Value=Gamma4
  Gamma5 : Constant  Value=Gamma5
  Gamma6 : Constant  Value=Gamma6
  Gamma7 : Constant  Value=Gamma6
  Gamma8 : Constant  Value=Gamma8
  Gamma9 : Constant  Value=Gamma9
  Mux3 : Mux  Inputs=11
  Gamma : Outport
  wires:
  Gamma9/1 -> Mux3/9
  Gamma6/1 -> Mux3/6
  Mux3/1 -> Gamma/1
  Gamma8/1 -> Mux3/8
  Gamma5/1 -> Mux3/5
  Gamma7/1 -> Mux3/7
  Gamma4/1 -> Mux3/4
  Gamma3/1 -> Mux3/3
  Gamma2/1 -> Mux3/2
  Gamma1/1 -> Mux3/1
  Gamma10/1 -> Mux3/10
  Gamma11/1 -> Mux3/11

== system Quad_Nonlinear_Roll_PS/Quadcopter 3DOF Nonlinear System4/Quad System/Quad System/dot(x1) ==
  X : Inport
  1 : Subsystem
  Add : Sum  Inputs=+++
  Subsystem : Subsystem
  Subsystem1 : Subsystem
  dot(x1) : Outport
  wires:
  X/1 -> Subsystem1/1(X), Subsystem/1(X), 1/1(X)  "X"
  Subsystem1/1(x4) -> Add/3
  Subsystem/1(x6cos(x1)tan(x2)) -> Add/2
  Add/1 -> dot(x1)/1
  1/1(x5sin(x1)tan(x2)) -> Add/1

== system Quad_Nonlinear_Roll_PS/Quadcopter 3DOF Nonlinear System4/Quad System/Quad System/dot(x2) ==
  X : Inport
  1 : Subsystem
  Add : Sum  Inputs=+-
  Subsystem : Subsystem
  dot(x2) : Outport
  wires:
  X/1 -> Subsystem/1(X), 1/1(X)  "X"
  Subsystem/1(x6sin(x1)) -> Add/2
  Add/1 -> dot(x2)/1
  1/1(x5cos(x1)) -> Add/1

== system Quad_Nonlinear_Roll_PS/Quadcopter 3DOF Nonlinear System4/Quad System/Quad System/dot(x3) ==
  X : Inport
  1 : Subsystem
  Add : Sum
  Product : Product
  Subsystem : Subsystem
  Subsystem1 : Subsystem
  dot(x3) : Outport
  wires:
  X/1 -> Subsystem1/1(X), Subsystem/1(X), 1/1(X)  "X"
  Subsystem/1(x6cos(x1)) -> Add/2
  1/1(x5sin(x1)) -> Add/1
  Product/1 -> dot(x3)/1
  Add/1 -> Product/1
  Subsystem1/1(sec(x2)) -> Product/2

== system Quad_Nonlinear_Roll_PS/Quadcopter 3DOF Nonlinear System/Quad System/Quad System/dot(x1)/1 ==
  X : Inport
  Demux : Demux  Outputs=6
  Subsystem : Subsystem
  Terminator : Terminator
  Terminator1 : Terminator
  Terminator2 : Terminator
  x5sin(x1)tan(x2) : Outport
  wires:
  Demux/2 -> Subsystem/2(x2)  "x2"
  Demux/4 -> Terminator1/1  "x4"
  X/1 -> Demux/1  "x"
  Demux/1 -> Subsystem/1(x1)  "x1"
  Demux/3 -> Terminator/1  "x3"
  Demux/6 -> Terminator2/1  "x6"
  Demux/5 -> Subsystem/3(x5)  "x5"
  Subsystem/1(x5sin(x1)tan(x2)) -> x5sin(x1)tan(x2)/1

== system Quad_Nonlinear_Roll_PS/Quadcopter 3DOF Nonlinear System/Quad System/Quad System/dot(x1)/Subsystem ==
  X : Inport
  Demux : Demux  Outputs=6
  Subsystem1 : Subsystem
  Terminator : Terminator
  Terminator1 : Terminator
  Terminator3 : Terminator
  x6cos(x1)tan(x2) : Outport
  wires:
  Demux/1 -> Subsystem1/1(x1)  "x1"
  Demux/3 -> Terminator/1  "x3"
  Demux/4 -> Terminator1/1  "x4"
  Demux/5 -> Terminator3/1  "x5"
  Demux/6 -> Subsystem1/3(x6)  "x6"
  Subsystem1/1(x6cos(x1)tan(x2)) -> x6cos(x1)tan(x2)/1  "x6cos(x1)tan(x2)"
  X/1 -> Demux/1  "X"
  Demux/2 -> Subsystem1/2(x2)  "x2"

== system Quad_Nonlinear_Roll_PS/Quadcopter 3DOF Nonlinear System/Quad System/Quad System/dot(x1)/Subsystem1 ==
  X : Inport
  Demux : Demux  Outputs=6
  Terminator{,2..5} (5 alike) : Terminator
  x4 : Outport
  wires:
  Demux/6 -> Terminator5/1  "x6"
  X/1 -> Demux/1
  Demux/3 -> Terminator/1  "x3"
  Demux/1 -> Terminator4/1  "x1"
  Demux/2 -> Terminator2/1  "x2"
  Demux/5 -> Terminator3/1  "x5"
  Demux/4 -> x4/1  "x4"

== system Quad_Nonlinear_Roll_PS/Quadcopter 3DOF Nonlinear System/Quad System/Quad System/dot(x2)/1 ==
  X : Inport
  Demux : Demux  Outputs=6
  Subsystem : Subsystem
  Terminator{,1..3} (4 alike) : Terminator
  x5cos(x1) : Outport
  wires:
  Demux/4 -> Terminator1/1  "x4"
  X/1 -> Demux/1  "x"
  Demux/1 -> Subsystem/1(x1)  "x1"
  Demux/3 -> Terminator/1  "x3"
  Demux/6 -> Terminator2/1  "x6"
  Demux/5 -> Subsystem/2(x5)  "x5"
  Subsystem/1(Out1) -> x5cos(x1)/1
  Demux/2 -> Terminator3/1  "x2"

== system Quad_Nonlinear_Roll_PS/Quadcopter 3DOF Nonlinear System/Quad System/Quad System/dot(x2)/Subsystem ==
  X : Inport
  Demux : Demux  Outputs=6
  Subsystem1 : Subsystem
  Terminator{,1..3} (4 alike) : Terminator
  x6sin(x1) : Outport
  wires:
  Demux/1 -> Subsystem1/1(x1)  "x1"
  Demux/3 -> Terminator/1  "x3"
  Demux/4 -> Terminator1/1  "x4"
  Demux/5 -> Terminator3/1  "x5"
  Demux/6 -> Subsystem1/2(x6)  "x6"
  Subsystem1/1(Out1) -> x6sin(x1)/1  "x6sin(x1)"
  X/1 -> Demux/1  "X"
  Demux/2 -> Terminator2/1  "x2"

== system Quad_Nonlinear_Roll_PS/Quadcopter 3DOF Nonlinear System/Quad System/Quad System/dot(x3)/1 ==
  X : Inport
  Demux : Demux  Outputs=6
  Subsystem : Subsystem
  Terminator{,1..3} (4 alike) : Terminator
  x5sin(x1) : Outport
  wires:
  Demux/4 -> Terminator1/1  "x4"
  X/1 -> Demux/1  "x"
  Demux/1 -> Subsystem/1(x1)  "x1"
  Demux/3 -> Terminator/1  "x3"
  Demux/6 -> Terminator2/1  "x6"
  Demux/5 -> Subsystem/2(x5)  "x5"
  Subsystem/1(x5sin(x1)) -> x5sin(x1)/1
  Demux/2 -> Terminator3/1  "x2"

== system Quad_Nonlinear_Roll_PS/Quadcopter 3DOF Nonlinear System/Quad System/Quad System/dot(x3)/Subsystem ==
  X : Inport
  Demux : Demux  Outputs=6
  Subsystem1 : Subsystem
  Terminator{,1..3} (4 alike) : Terminator
  x6cos(x1) : Outport
  wires:
  Demux/1 -> Subsystem1/1(x1)  "x1"
  Demux/3 -> Terminator/1  "x3"
  Demux/4 -> Terminator1/1  "x4"
  Demux/5 -> Terminator3/1  "x5"
  Demux/6 -> Subsystem1/2(x6)  "x6"
  Subsystem1/1(Out1) -> x6cos(x1)/1  "x6cos(x1)"
  X/1 -> Demux/1  "X"
  Demux/2 -> Terminator2/1  "x2"

== system Quad_Nonlinear_Roll_PS/Quadcopter 3DOF Nonlinear System/Quad System/Quad System/dot(x3)/Subsystem1 ==
  X : Inport
  Demux : Demux  Outputs=6
  Sec : Subsystem
  Terminator{,1..4} (5 alike) : Terminator
  sec(x2) : Outport
  wires:
  Demux/3 -> Terminator/1  "x3"
  Demux/4 -> Terminator1/1  "x4"
  Demux/5 -> Terminator3/1  "x5"
  X/1 -> Demux/1  "X"
  Demux/1 -> Terminator2/1  "x1"
  Demux/6 -> Terminator4/1  "x6"
  Demux/2 -> Sec/1(x2)  "x2"
  Sec/1(Sec(x2)) -> sec(x2)/1

== system Quad_Nonlinear_Roll_PS/Quadcopter 3DOF Nonlinear System1/Quad System/Quad System/dot(x1)/1 ==
  X : Inport
  Demux : Demux  Outputs=6
  Subsystem : Subsystem
  Terminator : Terminator
  Terminator1 : Terminator
  Terminator2 : Terminator
  x5sin(x1)tan(x2) : Outport
  wires:
  Demux/2 -> Subsystem/2(x2)  "x2"
  Demux/4 -> Terminator1/1  "x4"
  X/1 -> Demux/1  "x"
  Demux/1 -> Subsystem/1(x1)  "x1"
  Demux/3 -> Terminator/1  "x3"
  Demux/6 -> Terminator2/1  "x6"
  Demux/5 -> Subsystem/3(x5)  "x5"
  Subsystem/1(x5sin(x1)tan(x2)) -> x5sin(x1)tan(x2)/1

== system Quad_Nonlinear_Roll_PS/Quadcopter 3DOF Nonlinear System1/Quad System/Quad System/dot(x1)/Subsystem ==
  X : Inport
  Demux : Demux  Outputs=6
  Subsystem1 : Subsystem
  Terminator : Terminator
  Terminator1 : Terminator
  Terminator3 : Terminator
  x6cos(x1)tan(x2) : Outport
  wires:
  Demux/1 -> Subsystem1/1(x1)  "x1"
  Demux/3 -> Terminator/1  "x3"
  Demux/4 -> Terminator1/1  "x4"
  Demux/5 -> Terminator3/1  "x5"
  Demux/6 -> Subsystem1/3(x6)  "x6"
  Subsystem1/1(x6cos(x1)tan(x2)) -> x6cos(x1)tan(x2)/1  "x6cos(x1)tan(x2)"
  X/1 -> Demux/1  "X"
  Demux/2 -> Subsystem1/2(x2)  "x2"

== system Quad_Nonlinear_Roll_PS/Quadcopter 3DOF Nonlinear System1/Quad System/Quad System/dot(x1)/Subsystem1 ==
  X : Inport
  Demux : Demux  Outputs=6
  Terminator{,2..5} (5 alike) : Terminator
  x4 : Outport
  wires:
  Demux/6 -> Terminator5/1  "x6"
  X/1 -> Demux/1
  Demux/3 -> Terminator/1  "x3"
  Demux/1 -> Terminator4/1  "x1"
  Demux/2 -> Terminator2/1  "x2"
  Demux/5 -> Terminator3/1  "x5"
  Demux/4 -> x4/1  "x4"

== system Quad_Nonlinear_Roll_PS/Quadcopter 3DOF Nonlinear System1/Quad System/Quad System/dot(x2)/1 ==
  X : Inport
  Demux : Demux  Outputs=6
  Subsystem : Subsystem
  Terminator{,1..3} (4 alike) : Terminator
  x5cos(x1) : Outport
  wires:
  Demux/4 -> Terminator1/1  "x4"
  X/1 -> Demux/1  "x"
  Demux/1 -> Subsystem/1(x1)  "x1"
  Demux/3 -> Terminator/1  "x3"
  Demux/6 -> Terminator2/1  "x6"
  Demux/5 -> Subsystem/2(x5)  "x5"
  Subsystem/1(Out1) -> x5cos(x1)/1
  Demux/2 -> Terminator3/1  "x2"

== system Quad_Nonlinear_Roll_PS/Quadcopter 3DOF Nonlinear System1/Quad System/Quad System/dot(x2)/Subsystem ==
  X : Inport
  Demux : Demux  Outputs=6
  Subsystem1 : Subsystem
  Terminator{,1..3} (4 alike) : Terminator
  x6sin(x1) : Outport
  wires:
  Demux/1 -> Subsystem1/1(x1)  "x1"
  Demux/3 -> Terminator/1  "x3"
  Demux/4 -> Terminator1/1  "x4"
  Demux/5 -> Terminator3/1  "x5"
  Demux/6 -> Subsystem1/2(x6)  "x6"
  Subsystem1/1(Out1) -> x6sin(x1)/1  "x6sin(x1)"
  X/1 -> Demux/1  "X"
  Demux/2 -> Terminator2/1  "x2"

== system Quad_Nonlinear_Roll_PS/Quadcopter 3DOF Nonlinear System1/Quad System/Quad System/dot(x3)/1 ==
  X : Inport
  Demux : Demux  Outputs=6
  Subsystem : Subsystem
  Terminator{,1..3} (4 alike) : Terminator
  x5sin(x1) : Outport
  wires:
  Demux/4 -> Terminator1/1  "x4"
  X/1 -> Demux/1  "x"
  Demux/1 -> Subsystem/1(x1)  "x1"
  Demux/3 -> Terminator/1  "x3"
  Demux/6 -> Terminator2/1  "x6"
  Demux/5 -> Subsystem/2(x5)  "x5"
  Subsystem/1(x5sin(x1)) -> x5sin(x1)/1
  Demux/2 -> Terminator3/1  "x2"

== system Quad_Nonlinear_Roll_PS/Quadcopter 3DOF Nonlinear System1/Quad System/Quad System/dot(x3)/Subsystem ==
  X : Inport
  Demux : Demux  Outputs=6
  Subsystem1 : Subsystem
  Terminator{,1..3} (4 alike) : Terminator
  x6cos(x1) : Outport
  wires:
  Demux/1 -> Subsystem1/1(x1)  "x1"
  Demux/3 -> Terminator/1  "x3"
  Demux/4 -> Terminator1/1  "x4"
  Demux/5 -> Terminator3/1  "x5"
  Demux/6 -> Subsystem1/2(x6)  "x6"
  Subsystem1/1(Out1) -> x6cos(x1)/1  "x6cos(x1)"
  X/1 -> Demux/1  "X"
  Demux/2 -> Terminator2/1  "x2"

== system Quad_Nonlinear_Roll_PS/Quadcopter 3DOF Nonlinear System1/Quad System/Quad System/dot(x3)/Subsystem1 ==
  X : Inport
  Demux : Demux  Outputs=6
  Sec : Subsystem
  Terminator{,1..4} (5 alike) : Terminator
  sec(x2) : Outport
  wires:
  Demux/3 -> Terminator/1  "x3"
  Demux/4 -> Terminator1/1  "x4"
  Demux/5 -> Terminator3/1  "x5"
  X/1 -> Demux/1  "X"
  Demux/1 -> Terminator2/1  "x1"
  Demux/6 -> Terminator4/1  "x6"
  Demux/2 -> Sec/1(x2)  "x2"
  Sec/1(Sec(x2)) -> sec(x2)/1

== system Quad_Nonlinear_Roll_PS/Quadcopter 3DOF Nonlinear System2/Quad System/Quad System/dot(x1)/1 ==
  X : Inport
  Demux : Demux  Outputs=6
  Subsystem : Subsystem
  Terminator : Terminator
  Terminator1 : Terminator
  Terminator2 : Terminator
  x5sin(x1)tan(x2) : Outport
  wires:
  Demux/2 -> Subsystem/2(x2)  "x2"
  Demux/4 -> Terminator1/1  "x4"
  X/1 -> Demux/1  "x"
  Demux/1 -> Subsystem/1(x1)  "x1"
  Demux/3 -> Terminator/1  "x3"
  Demux/6 -> Terminator2/1  "x6"
  Demux/5 -> Subsystem/3(x5)  "x5"
  Subsystem/1(x5sin(x1)tan(x2)) -> x5sin(x1)tan(x2)/1

== system Quad_Nonlinear_Roll_PS/Quadcopter 3DOF Nonlinear System2/Quad System/Quad System/dot(x1)/Subsystem ==
  X : Inport
  Demux : Demux  Outputs=6
  Subsystem1 : Subsystem
  Terminator : Terminator
  Terminator1 : Terminator
  Terminator3 : Terminator
  x6cos(x1)tan(x2) : Outport
  wires:
  Demux/1 -> Subsystem1/1(x1)  "x1"
  Demux/3 -> Terminator/1  "x3"
  Demux/4 -> Terminator1/1  "x4"
  Demux/5 -> Terminator3/1  "x5"
  Demux/6 -> Subsystem1/3(x6)  "x6"
  Subsystem1/1(x6cos(x1)tan(x2)) -> x6cos(x1)tan(x2)/1  "x6cos(x1)tan(x2)"
  X/1 -> Demux/1  "X"
  Demux/2 -> Subsystem1/2(x2)  "x2"

== system Quad_Nonlinear_Roll_PS/Quadcopter 3DOF Nonlinear System2/Quad System/Quad System/dot(x1)/Subsystem1 ==
  X : Inport
  Demux : Demux  Outputs=6
  Terminator{,2..5} (5 alike) : Terminator
  x4 : Outport
  wires:
  Demux/6 -> Terminator5/1  "x6"
  X/1 -> Demux/1
  Demux/3 -> Terminator/1  "x3"
  Demux/1 -> Terminator4/1  "x1"
  Demux/2 -> Terminator2/1  "x2"
  Demux/5 -> Terminator3/1  "x5"
  Demux/4 -> x4/1  "x4"

== system Quad_Nonlinear_Roll_PS/Quadcopter 3DOF Nonlinear System2/Quad System/Quad System/dot(x2)/1 ==
  X : Inport
  Demux : Demux  Outputs=6
  Subsystem : Subsystem
  Terminator{,1..3} (4 alike) : Terminator
  x5cos(x1) : Outport
  wires:
  Demux/4 -> Terminator1/1  "x4"
  X/1 -> Demux/1  "x"
  Demux/1 -> Subsystem/1(x1)  "x1"
  Demux/3 -> Terminator/1  "x3"
  Demux/6 -> Terminator2/1  "x6"
  Demux/5 -> Subsystem/2(x5)  "x5"
  Subsystem/1(Out1) -> x5cos(x1)/1
  Demux/2 -> Terminator3/1  "x2"

== system Quad_Nonlinear_Roll_PS/Quadcopter 3DOF Nonlinear System2/Quad System/Quad System/dot(x2)/Subsystem ==
  X : Inport
  Demux : Demux  Outputs=6
  Subsystem1 : Subsystem
  Terminator{,1..3} (4 alike) : Terminator
  x6sin(x1) : Outport
  wires:
  Demux/1 -> Subsystem1/1(x1)  "x1"
  Demux/3 -> Terminator/1  "x3"
  Demux/4 -> Terminator1/1  "x4"
  Demux/5 -> Terminator3/1  "x5"
  Demux/6 -> Subsystem1/2(x6)  "x6"
  Subsystem1/1(Out1) -> x6sin(x1)/1  "x6sin(x1)"
  X/1 -> Demux/1  "X"
  Demux/2 -> Terminator2/1  "x2"

== system Quad_Nonlinear_Roll_PS/Quadcopter 3DOF Nonlinear System2/Quad System/Quad System/dot(x3)/1 ==
  X : Inport
  Demux : Demux  Outputs=6
  Subsystem : Subsystem
  Terminator{,1..3} (4 alike) : Terminator
  x5sin(x1) : Outport
  wires:
  Demux/4 -> Terminator1/1  "x4"
  X/1 -> Demux/1  "x"
  Demux/1 -> Subsystem/1(x1)  "x1"
  Demux/3 -> Terminator/1  "x3"
  Demux/6 -> Terminator2/1  "x6"
  Demux/5 -> Subsystem/2(x5)  "x5"
  Subsystem/1(x5sin(x1)) -> x5sin(x1)/1
  Demux/2 -> Terminator3/1  "x2"

== system Quad_Nonlinear_Roll_PS/Quadcopter 3DOF Nonlinear System2/Quad System/Quad System/dot(x3)/Subsystem ==
  X : Inport
  Demux : Demux  Outputs=6
  Subsystem1 : Subsystem
  Terminator{,1..3} (4 alike) : Terminator
  x6cos(x1) : Outport
  wires:
  Demux/1 -> Subsystem1/1(x1)  "x1"
  Demux/3 -> Terminator/1  "x3"
  Demux/4 -> Terminator1/1  "x4"
  Demux/5 -> Terminator3/1  "x5"
  Demux/6 -> Subsystem1/2(x6)  "x6"
  Subsystem1/1(Out1) -> x6cos(x1)/1  "x6cos(x1)"
  X/1 -> Demux/1  "X"
  Demux/2 -> Terminator2/1  "x2"

== system Quad_Nonlinear_Roll_PS/Quadcopter 3DOF Nonlinear System2/Quad System/Quad System/dot(x3)/Subsystem1 ==
  X : Inport
  Demux : Demux  Outputs=6
  Sec : Subsystem
  Terminator{,1..4} (5 alike) : Terminator
  sec(x2) : Outport
  wires:
  Demux/3 -> Terminator/1  "x3"
  Demux/4 -> Terminator1/1  "x4"
  Demux/5 -> Terminator3/1  "x5"
  X/1 -> Demux/1  "X"
  Demux/1 -> Terminator2/1  "x1"
  Demux/6 -> Terminator4/1  "x6"
  Demux/2 -> Sec/1(x2)  "x2"
  Sec/1(Sec(x2)) -> sec(x2)/1

== system Quad_Nonlinear_Roll_PS/Quadcopter 3DOF Nonlinear System3/Quad System/Quad System/dot(x1)/1 ==
  X : Inport
  Demux : Demux  Outputs=6
  Subsystem : Subsystem
  Terminator : Terminator
  Terminator1 : Terminator
  Terminator2 : Terminator
  x5sin(x1)tan(x2) : Outport
  wires:
  Demux/2 -> Subsystem/2(x2)  "x2"
  Demux/4 -> Terminator1/1  "x4"
  X/1 -> Demux/1  "x"
  Demux/1 -> Subsystem/1(x1)  "x1"
  Demux/3 -> Terminator/1  "x3"
  Demux/6 -> Terminator2/1  "x6"
  Demux/5 -> Subsystem/3(x5)  "x5"
  Subsystem/1(x5sin(x1)tan(x2)) -> x5sin(x1)tan(x2)/1

== system Quad_Nonlinear_Roll_PS/Quadcopter 3DOF Nonlinear System3/Quad System/Quad System/dot(x1)/Subsystem ==
  X : Inport
  Demux : Demux  Outputs=6
  Subsystem1 : Subsystem
  Terminator : Terminator
  Terminator1 : Terminator
  Terminator3 : Terminator
  x6cos(x1)tan(x2) : Outport
  wires:
  Demux/1 -> Subsystem1/1(x1)  "x1"
  Demux/3 -> Terminator/1  "x3"
  Demux/4 -> Terminator1/1  "x4"
  Demux/5 -> Terminator3/1  "x5"
  Demux/6 -> Subsystem1/3(x6)  "x6"
  Subsystem1/1(x6cos(x1)tan(x2)) -> x6cos(x1)tan(x2)/1  "x6cos(x1)tan(x2)"
  X/1 -> Demux/1  "X"
  Demux/2 -> Subsystem1/2(x2)  "x2"

== system Quad_Nonlinear_Roll_PS/Quadcopter 3DOF Nonlinear System3/Quad System/Quad System/dot(x1)/Subsystem1 ==
  X : Inport
  Demux : Demux  Outputs=6
  Terminator{,2..5} (5 alike) : Terminator
  x4 : Outport
  wires:
  Demux/6 -> Terminator5/1  "x6"
  X/1 -> Demux/1
  Demux/3 -> Terminator/1  "x3"
  Demux/1 -> Terminator4/1  "x1"
  Demux/2 -> Terminator2/1  "x2"
  Demux/5 -> Terminator3/1  "x5"
  Demux/4 -> x4/1  "x4"

== system Quad_Nonlinear_Roll_PS/Quadcopter 3DOF Nonlinear System3/Quad System/Quad System/dot(x2)/1 ==
  X : Inport
  Demux : Demux  Outputs=6
  Subsystem : Subsystem
  Terminator{,1..3} (4 alike) : Terminator
  x5cos(x1) : Outport
  wires:
  Demux/4 -> Terminator1/1  "x4"
  X/1 -> Demux/1  "x"
  Demux/1 -> Subsystem/1(x1)  "x1"
  Demux/3 -> Terminator/1  "x3"
  Demux/6 -> Terminator2/1  "x6"
  Demux/5 -> Subsystem/2(x5)  "x5"
  Subsystem/1(Out1) -> x5cos(x1)/1
  Demux/2 -> Terminator3/1  "x2"

== system Quad_Nonlinear_Roll_PS/Quadcopter 3DOF Nonlinear System3/Quad System/Quad System/dot(x2)/Subsystem ==
  X : Inport
  Demux : Demux  Outputs=6
  Subsystem1 : Subsystem
  Terminator{,1..3} (4 alike) : Terminator
  x6sin(x1) : Outport
  wires:
  Demux/1 -> Subsystem1/1(x1)  "x1"
  Demux/3 -> Terminator/1  "x3"
  Demux/4 -> Terminator1/1  "x4"
  Demux/5 -> Terminator3/1  "x5"
  Demux/6 -> Subsystem1/2(x6)  "x6"
  Subsystem1/1(Out1) -> x6sin(x1)/1  "x6sin(x1)"
  X/1 -> Demux/1  "X"
  Demux/2 -> Terminator2/1  "x2"

== system Quad_Nonlinear_Roll_PS/Quadcopter 3DOF Nonlinear System3/Quad System/Quad System/dot(x3)/1 ==
  X : Inport
  Demux : Demux  Outputs=6
  Subsystem : Subsystem
  Terminator{,1..3} (4 alike) : Terminator
  x5sin(x1) : Outport
  wires:
  Demux/4 -> Terminator1/1  "x4"
  X/1 -> Demux/1  "x"
  Demux/1 -> Subsystem/1(x1)  "x1"
  Demux/3 -> Terminator/1  "x3"
  Demux/6 -> Terminator2/1  "x6"
  Demux/5 -> Subsystem/2(x5)  "x5"
  Subsystem/1(x5sin(x1)) -> x5sin(x1)/1
  Demux/2 -> Terminator3/1  "x2"

== system Quad_Nonlinear_Roll_PS/Quadcopter 3DOF Nonlinear System3/Quad System/Quad System/dot(x3)/Subsystem ==
  X : Inport
  Demux : Demux  Outputs=6
  Subsystem1 : Subsystem
  Terminator{,1..3} (4 alike) : Terminator
  x6cos(x1) : Outport
  wires:
  Demux/1 -> Subsystem1/1(x1)  "x1"
  Demux/3 -> Terminator/1  "x3"
  Demux/4 -> Terminator1/1  "x4"
  Demux/5 -> Terminator3/1  "x5"
  Demux/6 -> Subsystem1/2(x6)  "x6"
  Subsystem1/1(Out1) -> x6cos(x1)/1  "x6cos(x1)"
  X/1 -> Demux/1  "X"
  Demux/2 -> Terminator2/1  "x2"

== system Quad_Nonlinear_Roll_PS/Quadcopter 3DOF Nonlinear System3/Quad System/Quad System/dot(x3)/Subsystem1 ==
  X : Inport
  Demux : Demux  Outputs=6
  Sec : Subsystem
  Terminator{,1..4} (5 alike) : Terminator
  sec(x2) : Outport
  wires:
  Demux/3 -> Terminator/1  "x3"
  Demux/4 -> Terminator1/1  "x4"
  Demux/5 -> Terminator3/1  "x5"
  X/1 -> Demux/1  "X"
  Demux/1 -> Terminator2/1  "x1"
  Demux/6 -> Terminator4/1  "x6"
  Demux/2 -> Sec/1(x2)  "x2"
  Sec/1(Sec(x2)) -> sec(x2)/1

== system Quad_Nonlinear_Roll_PS/Quadcopter 3DOF Nonlinear System4/Quad System/Quad System/dot(x1)/1 ==
  X : Inport
  Demux : Demux  Outputs=6
  Subsystem : Subsystem
  Terminator : Terminator
  Terminator1 : Terminator
  Terminator2 : Terminator
  x5sin(x1)tan(x2) : Outport
  wires:
  Demux/2 -> Subsystem/2(x2)  "x2"
  Demux/4 -> Terminator1/1  "x4"
  X/1 -> Demux/1  "x"
  Demux/1 -> Subsystem/1(x1)  "x1"
  Demux/3 -> Terminator/1  "x3"
  Demux/6 -> Terminator2/1  "x6"
  Demux/5 -> Subsystem/3(x5)  "x5"
  Subsystem/1(x5sin(x1)tan(x2)) -> x5sin(x1)tan(x2)/1

== system Quad_Nonlinear_Roll_PS/Quadcopter 3DOF Nonlinear System4/Quad System/Quad System/dot(x1)/Subsystem ==
  X : Inport
  Demux : Demux  Outputs=6
  Subsystem1 : Subsystem
  Terminator : Terminator
  Terminator1 : Terminator
  Terminator3 : Terminator
  x6cos(x1)tan(x2) : Outport
  wires:
  Demux/1 -> Subsystem1/1(x1)  "x1"
  Demux/3 -> Terminator/1  "x3"
  Demux/4 -> Terminator1/1  "x4"
  Demux/5 -> Terminator3/1  "x5"
  Demux/6 -> Subsystem1/3(x6)  "x6"
  Subsystem1/1(x6cos(x1)tan(x2)) -> x6cos(x1)tan(x2)/1  "x6cos(x1)tan(x2)"
  X/1 -> Demux/1  "X"
  Demux/2 -> Subsystem1/2(x2)  "x2"

== system Quad_Nonlinear_Roll_PS/Quadcopter 3DOF Nonlinear System4/Quad System/Quad System/dot(x1)/Subsystem1 ==
  X : Inport
  Demux : Demux  Outputs=6
  Terminator{,2..5} (5 alike) : Terminator
  x4 : Outport
  wires:
  Demux/6 -> Terminator5/1  "x6"
  X/1 -> Demux/1
  Demux/3 -> Terminator/1  "x3"
  Demux/1 -> Terminator4/1  "x1"
  Demux/2 -> Terminator2/1  "x2"
  Demux/5 -> Terminator3/1  "x5"
  Demux/4 -> x4/1  "x4"

== system Quad_Nonlinear_Roll_PS/Quadcopter 3DOF Nonlinear System4/Quad System/Quad System/dot(x2)/1 ==
  X : Inport
  Demux : Demux  Outputs=6
  Subsystem : Subsystem
  Terminator{,1..3} (4 alike) : Terminator
  x5cos(x1) : Outport
  wires:
  Demux/4 -> Terminator1/1  "x4"
  X/1 -> Demux/1  "x"
  Demux/1 -> Subsystem/1(x1)  "x1"
  Demux/3 -> Terminator/1  "x3"
  Demux/6 -> Terminator2/1  "x6"
  Demux/5 -> Subsystem/2(x5)  "x5"
  Subsystem/1(Out1) -> x5cos(x1)/1
  Demux/2 -> Terminator3/1  "x2"

== system Quad_Nonlinear_Roll_PS/Quadcopter 3DOF Nonlinear System4/Quad System/Quad System/dot(x2)/Subsystem ==
  X : Inport
  Demux : Demux  Outputs=6
  Subsystem1 : Subsystem
  Terminator{,1..3} (4 alike) : Terminator
  x6sin(x1) : Outport
  wires:
  Demux/1 -> Subsystem1/1(x1)  "x1"
  Demux/3 -> Terminator/1  "x3"
  Demux/4 -> Terminator1/1  "x4"
  Demux/5 -> Terminator3/1  "x5"
  Demux/6 -> Subsystem1/2(x6)  "x6"
  Subsystem1/1(Out1) -> x6sin(x1)/1  "x6sin(x1)"
  X/1 -> Demux/1  "X"
  Demux/2 -> Terminator2/1  "x2"

== system Quad_Nonlinear_Roll_PS/Quadcopter 3DOF Nonlinear System4/Quad System/Quad System/dot(x3)/1 ==
  X : Inport
  Demux : Demux  Outputs=6
  Subsystem : Subsystem
  Terminator{,1..3} (4 alike) : Terminator
  x5sin(x1) : Outport
  wires:
  Demux/4 -> Terminator1/1  "x4"
  X/1 -> Demux/1  "x"
  Demux/1 -> Subsystem/1(x1)  "x1"
  Demux/3 -> Terminator/1  "x3"
  Demux/6 -> Terminator2/1  "x6"
  Demux/5 -> Subsystem/2(x5)  "x5"
  Subsystem/1(x5sin(x1)) -> x5sin(x1)/1
  Demux/2 -> Terminator3/1  "x2"

== system Quad_Nonlinear_Roll_PS/Quadcopter 3DOF Nonlinear System4/Quad System/Quad System/dot(x3)/Subsystem ==
  X : Inport
  Demux : Demux  Outputs=6
  Subsystem1 : Subsystem
  Terminator{,1..3} (4 alike) : Terminator
  x6cos(x1) : Outport
  wires:
  Demux/1 -> Subsystem1/1(x1)  "x1"
  Demux/3 -> Terminator/1  "x3"
  Demux/4 -> Terminator1/1  "x4"
  Demux/5 -> Terminator3/1  "x5"
  Demux/6 -> Subsystem1/2(x6)  "x6"
  Subsystem1/1(Out1) -> x6cos(x1)/1  "x6cos(x1)"
  X/1 -> Demux/1  "X"
  Demux/2 -> Terminator2/1  "x2"

== system Quad_Nonlinear_Roll_PS/Quadcopter 3DOF Nonlinear System4/Quad System/Quad System/dot(x3)/Subsystem1 ==
  X : Inport
  Demux : Demux  Outputs=6
  Sec : Subsystem
  Terminator{,1..4} (5 alike) : Terminator
  sec(x2) : Outport
  wires:
  Demux/3 -> Terminator/1  "x3"
  Demux/4 -> Terminator1/1  "x4"
  Demux/5 -> Terminator3/1  "x5"
  X/1 -> Demux/1  "X"
  Demux/1 -> Terminator2/1  "x1"
  Demux/6 -> Terminator4/1  "x6"
  Demux/2 -> Sec/1(x2)  "x2"
  Sec/1(Sec(x2)) -> sec(x2)/1

== system Quad_Nonlinear_Roll_PS/Quadcopter 3DOF Nonlinear System/Quad System/Quad System/dot(x1)/1/Subsystem ==
  x1 : Inport
  x2 : Inport  Port=2
  x5 : Inport  Port=3
  Product : Product  Inputs=3
  Sin : Trigonometry
  Tan : Trigonometry  Operator=tan
  x5sin(x1)tan(x2) : Outport
  wires:
  Sin/1 -> Product/1
  x5/1 -> Product/3
  Product/1 -> x5sin(x1)tan(x2)/1
  x1/1 -> Sin/1
  x2/1 -> Tan/1
  Tan/1 -> Product/2
